simulink model "Motor_Control"  (R2020a)
settings: Solver=VariableStepAuto  StartTime=0.0  StopTime=2  RelTol=1e-3
values from neighbouring files (symbols this model uses):
  b = 2.58984 * 10^(-5)    (= 2.58984e-05)    [MotorInformation.m]
  d = 0.15    [MotorInformation.m]
  J = (1/12)*(0.32^2+0.4^2)*M + M*0.15^2    (= 0.354933333333)    [MotorInformation.m]
  Kac = 1/Kpc    (= 0.0636619772368)    [MotorInformation.m]
  Kas = 1/(2.8*Kps)    (= 40.4186448067)    [MotorInformation.m]
  Ke = 0.0195    [MotorInformation.m]
  Kic = R * Wcc*1.3    (= 24504.422698)    [MotorInformation.m]
  Kis = Jm*Wcs^2/(Kt)    (= 2.77594011786)    [MotorInformation.m]
  Kpc = La * Wcc    (= 15.7079632679)    [MotorInformation.m]
  Kps = Jm * Wcs/Kt    (= 0.00883609182968)    [MotorInformation.m]
  Kt = 0.0195    [MotorInformation.m]
  L = 0.1655    [MotorInformation.m]
  La = 0.005    [MotorInformation.m]
  M = 8    [MotorInformation.m]
  n = 49    [MotorInformation.m]
  R = 6    [MotorInformation.m]
  Rw = 0.155/2    (= 0.0775)    [MotorInformation.m]
libraries: simulink x2
settings Model: Creator=hambi  LastModifiedBy=hambi

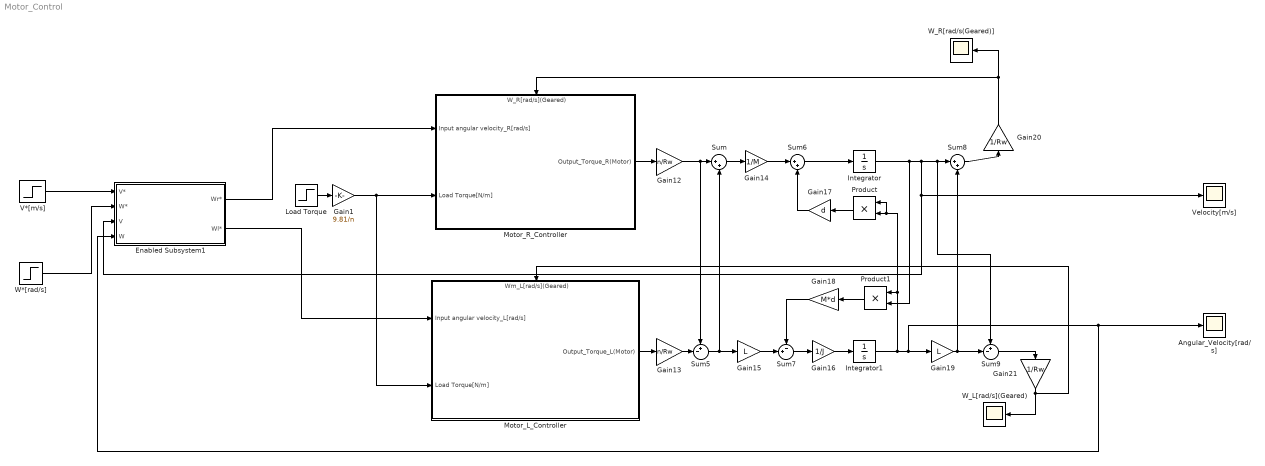
== system Motor_Control ==
  Angular_Velocity[rad/s] : Scope
  Enabled Subsystem1 : Subsystem  TreatAsAtomicUnit=on
  Gain1 : Gain  Gain=9.81/n
  Gain12 : Gain  Gain=n/Rw
  Gain13 : Gain  Gain=n/Rw
  Gain14 : Gain  Gain=1/M
  Gain15 : Gain  Gain=L
  Gain16 : Gain  Gain=1/J
  Gain17 : Gain  Gain=d
  Gain18 : Gain  Gain=M*d
  Gain19 : Gain  Gain=L
  Gain20 : Gain  Gain=1/Rw
  Gain21 : Gain  Gain=1/Rw
  Integrator : Integrator
  Integrator1 : Integrator
  Load Torque : Step  Time=5  After=0  SampleTime=0
  Motor_L_Controller : Subsystem  TreatAsAtomicUnit=on
      settings: PortSchema="{\"entries\":[{\"content\":{\"sides\":[{\"content\":{\"connectorIds\":[\"In1\",\"In2\"]},\"type\":\"ConnectorPlacement.EquallySpacedRectSide\",\"uuid\":\"38708cf0-fa5b-4525-8073-2ea034bbba89\"},{\"content\":{\"connectorIds\":[\"Out1\"],\"side\":\"RIGHT\"},\"type\":\"ConnectorPlacement.EquallySpacedRectSide\",\"uuid\":\"66c4a39b-21a9-4a0c-b844-f8b5c61f778e\"},{\"content\":{\"connectorIds\":[\"In3\"],\"side\":\"TOP\"},\"type\":\"ConnectorPlacement.EquallySpacedRectSide\",\"uuid\":\"4e6c23e5-8516-4ab2-b702-67db97948711\"}]},\"type\":\"ConnectorPlacement.EquallySpacedConnector\",\"uuid\":\"2dafcc4f-e74b-4b96-80e8-79cd761172ee\"}],\"packageUris\":[\"http://schema.mathworks.com/mf0/Connector/19700101\"],\"version\":\"1.0\"}"
  Motor_R_Controller : Subsystem  TreatAsAtomicUnit=on
      settings: PortSchema="{\"entries\":[{\"content\":{\"sides\":[{\"content\":{\"connectorIds\":[\"In1\",\"In2\"]},\"type\":\"ConnectorPlacement.EquallySpacedRectSide\",\"uuid\":\"38708cf0-fa5b-4525-8073-2ea034bbba89\"},{\"content\":{\"connectorIds\":[\"Out1\"],\"side\":\"RIGHT\"},\"type\":\"ConnectorPlacement.EquallySpacedRectSide\",\"uuid\":\"66c4a39b-21a9-4a0c-b844-f8b5c61f778e\"},{\"content\":{\"connectorIds\":[\"In3\"],\"side\":\"TOP\"},\"type\":\"ConnectorPlacement.EquallySpacedRectSide\",\"uuid\":\"4e6c23e5-8516-4ab2-b702-67db97948711\"}]},\"type\":\"ConnectorPlacement.EquallySpacedConnector\",\"uuid\":\"2dafcc4f-e74b-4b96-80e8-79cd761172ee\"}],\"packageUris\":[\"http://schema.mathworks.com/mf0/Connector/19700101\"],\"version\":\"1.0\"}"
  Product : Product
  Product1 : Product
  Sum : Sum  Inputs=|++
  Sum5 : Sum  Inputs=+-|
  Sum6 : Sum  Inputs=|++
  Sum7 : Sum  Inputs=-+|
  Sum8 : Sum  Inputs=|++
  Sum9 : Sum  Inputs=+-|
  V*[m/s] : Step  Time=0  After=0.20  SampleTime=0  ZeroCross=off
  Velocity[m/s] : Scope
  W*[rad/s] : Step  Time=0  After=0.028  SampleTime=0  ZeroCross=off
  W_L[rad/s](Geared) : Scope
  W_R[rad/s(Geared)] : Scope
  wires:
  Sum8/1 -> Gain20/1
  Gain20/1 -> Motor_R_Controller/3(W_R[rad/s](Geared)), W_R[rad/s(Geared)]/1
  Gain21/1 -> Motor_L_Controller/3(Wm_L[rad/s](Geared)), W_L[rad/s](Geared)/1
  Sum9/1 -> Gain21/1
  Product1/1 -> Gain18/1
  Product/1 -> Gain17/1
  Gain14/1 -> Sum6/1
  Gain16/1 -> Integrator1/1
  Motor_R_Controller/1(Output_Torque_R(Motor)) -> Gain12/1
  Integrator/1 -> Enabled Subsystem1/3(V), Velocity[m/s]/1, Sum9/1, Sum8/1, Product1/2
  Gain1/1 -> Motor_L_Controller/2(Load Torque[N/m]), Motor_R_Controller/2(Load Torque[N/m])
  Gain19/1 -> Sum9/2, Sum8/2
  Enabled Subsystem1/1(Wr*) -> Motor_R_Controller/1(Input angular velocity_R[rad/s])
  Motor_L_Controller/1(Output_Torque_L(Motor)) -> Gain13/1
  Gain13/1 -> Sum5/2
  Sum6/1 -> Integrator/1
  Sum7/1 -> Gain16/1
  Gain15/1 -> Sum7/2
  Gain18/1 -> Sum7/1
  Gain17/1 -> Sum6/2
  Gain12/1 -> Sum5/1, Sum/1
  Sum/1 -> Gain14/1
  Sum5/1 -> Gain15/1, Sum/2
  Load Torque/1 -> Gain1/1
  Integrator1/1 -> Angular_Velocity[rad/s]/1, Enabled Subsystem1/4(W), Gain19/1, Product/1, Product/2, Product1/1
  V*[m/s]/1 -> Enabled Subsystem1/1(V*)
  W*[rad/s]/1 -> Enabled Subsystem1/2(W*)
  Enabled Subsystem1/2(Wl*) -> Motor_L_Controller/1(Input angular velocity_L[rad/s])

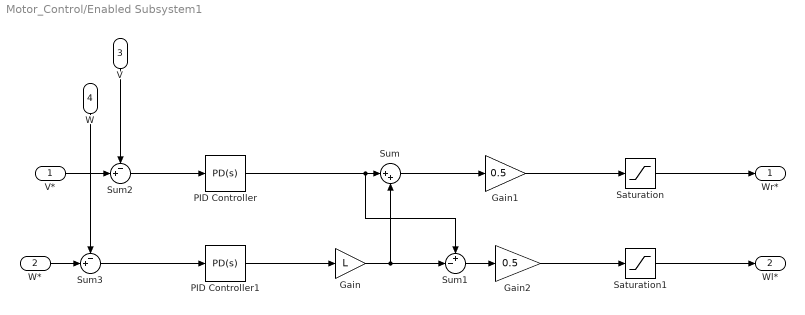
== system Motor_Control/Enabled Subsystem1 ==
  V* : Inport
  W* : Inport  Port=2
  V : Inport  Port=3
  W : Inport  Port=4
  Gain : Gain  Gain=L
  Gain1 : Gain  Gain=0.5
  Gain2 : Gain  Gain=0.5
  PID Controller : simulink/Continuous/PID Controller  Controller=PD  Form=Parallel  TimeDomain=Continuous-time  UseExternalTs=off  SampleTime=-1  IntegratorMethod=Forward Euler  FilterMethod=Forward Euler  ControllerParametersSource=internal  P=3.3  I=1  D=0.0145  UseFilter=on  N=100  TunerSelectOption=Transfer Function Based (PID Tuner App)  InitialConditionSource=internal  InitialConditionForIntegrator=0  InitialConditionForFilter=0  DifferentiatorICPrevScaledInput=0  ExternalReset=none  TrackingMode=off  Kt=1  LimitOutput=off  UpperSaturationLimit=inf  LowerSaturationLimit=-inf  LinearizeAsGain=on  AntiWindupMode=none  Kb=1  POutMin=[]  POutMax=[]  IOutMin=[]  IOutMax=[]  DOutMin=[]  DOutMax=[]  NOutMin=[]  NOutMax=[]  SumOutMin=[]  SumOutMax=[]  SaturationOutMin=[]  SaturationOutMax=[]  PParamMin=[]  PParamMax=[]  IParamMin=[]  IParamMax=[]  DParamMin=[]  DParamMax=[]  NParamMin=[]  NParamMax=[]  KbParamMin=[]  KbParamMax=[]  KtParamMin=[]  KtParamMax=[]  KbOutMin=[]  KbOutMax=[]  KtOutMin=[]  KtOutMax=[]  IntegratorOutMin=[]  IntegratorOutMax=[]  FilterOutMin=[]  FilterOutMax=[]  SumI1OutMin=[]  SumI1OutMax=[]  SumI2OutMin=[]  SumI2OutMax=[]  SumI3OutMin=[]  SumI3OutMax=[]  SumI4OutMin=[]  SumI4OutMax=[]  SumDOutMin=[]  SumDOutMax=[]  DifferentiatorOutMin=[]  DifferentiatorOutMax=[]  FilterDiffOutCoefMin=[]  FilterDiffOutCoefMax=[]  ReciprocalOutMin=[]  ReciprocalOutMax=[]  SumDenOutMin=[]  SumDenOutMax=[]  SumNumOutMin=[]  SumNumOutMax=[]  DivideOutMin=[]  DivideOutMax=[]  UdiffTsProdOutMin=[]  UdiffTsProdOutMax=[]  NTsProdOutMin=[]  NTsProdOutMax=[]  UintegralTsProdOutMin=[]  UintegralTsProdOutMax=[]  UngainTsProdOutMin=[]  UngainTsProdOutMax=[]  IntegratorContinuousStateAttributes=''  IntegratorStateMustResolveToSignalObject=off  IntegratorRTWStateStorageClass=Auto  FilterContinuousStateAttributes=''  FilterStateMustResolveToSignalObject=off  FilterRTWStateStorageClass=Auto  ParallelPVariant=InternalParameters  IdealPVariant=Disabled  IVariant=Disabled  DVariant=InternalParameters  IntegratorVariant=Disabled  SatVariant=Disabled  AWVariant=Disabled  PCopyVariant=Disabled  TRVariant=Disabled  FdbkBlocksVariant=Forward  IdealPFdbkVariant=Disabled  SatFdbkVariant=Disabled  DerivativeFilterVariant=ContFilter  NVariant=InternalParameters  NCopyVariant=Disabled  FilterICVariant=InternalICsFilter  IntegratorICVariant=Disabled  ExternalResetVariant=Disabled  TRSumVariant=Passthrough  SumFdbkVariant=Disabled  SumVariant=Sum_PD  TsampFilterVariant=InternalTs  TsampNgainVariant=Passthrough  TsampIntegralVariant=Disabled_SignalSpec
  PID Controller1 : simulink/Continuous/PID Controller  Controller=PD  Form=Parallel  TimeDomain=Continuous-time  UseExternalTs=off  SampleTime=-1  IntegratorMethod=Forward Euler  FilterMethod=Forward Euler  ControllerParametersSource=internal  P=5  I=1  D=0  UseFilter=on  N=100  TunerSelectOption=Transfer Function Based (PID Tuner App)  InitialConditionSource=internal  InitialConditionForIntegrator=0  InitialConditionForFilter=0  DifferentiatorICPrevScaledInput=0  ExternalReset=none  TrackingMode=off  Kt=1  LimitOutput=off  UpperSaturationLimit=inf  LowerSaturationLimit=-inf  LinearizeAsGain=on  AntiWindupMode=none  Kb=1  POutMin=[]  POutMax=[]  IOutMin=[]  IOutMax=[]  DOutMin=[]  DOutMax=[]  NOutMin=[]  NOutMax=[]  SumOutMin=[]  SumOutMax=[]  SaturationOutMin=[]  SaturationOutMax=[]  PParamMin=[]  PParamMax=[]  IParamMin=[]  IParamMax=[]  DParamMin=[]  DParamMax=[]  NParamMin=[]  NParamMax=[]  KbParamMin=[]  KbParamMax=[]  KtParamMin=[]  KtParamMax=[]  KbOutMin=[]  KbOutMax=[]  KtOutMin=[]  KtOutMax=[]  IntegratorOutMin=[]  IntegratorOutMax=[]  FilterOutMin=[]  FilterOutMax=[]  SumI1OutMin=[]  SumI1OutMax=[]  SumI2OutMin=[]  SumI2OutMax=[]  SumI3OutMin=[]  SumI3OutMax=[]  SumI4OutMin=[]  SumI4OutMax=[]  SumDOutMin=[]  SumDOutMax=[]  DifferentiatorOutMin=[]  DifferentiatorOutMax=[]  FilterDiffOutCoefMin=[]  FilterDiffOutCoefMax=[]  ReciprocalOutMin=[]  ReciprocalOutMax=[]  SumDenOutMin=[]  SumDenOutMax=[]  SumNumOutMin=[]  SumNumOutMax=[]  DivideOutMin=[]  DivideOutMax=[]  UdiffTsProdOutMin=[]  UdiffTsProdOutMax=[]  NTsProdOutMin=[]  NTsProdOutMax=[]  UintegralTsProdOutMin=[]  UintegralTsProdOutMax=[]  UngainTsProdOutMin=[]  UngainTsProdOutMax=[]  IntegratorContinuousStateAttributes=''  IntegratorStateMustResolveToSignalObject=off  IntegratorRTWStateStorageClass=Auto  FilterContinuousStateAttributes=''  FilterStateMustResolveToSignalObject=off  FilterRTWStateStorageClass=Auto  ParallelPVariant=InternalParameters  IdealPVariant=Disabled  IVariant=Disabled  DVariant=InternalParameters  IntegratorVariant=Disabled  SatVariant=Disabled  AWVariant=Disabled  PCopyVariant=Disabled  TRVariant=Disabled  FdbkBlocksVariant=Forward  IdealPFdbkVariant=Disabled  SatFdbkVariant=Disabled  DerivativeFilterVariant=ContFilter  NVariant=InternalParameters  NCopyVariant=Disabled  FilterICVariant=InternalICsFilter  IntegratorICVariant=Disabled  ExternalResetVariant=Disabled  TRSumVariant=Passthrough  SumFdbkVariant=Disabled  SumVariant=Sum_PD  TsampFilterVariant=InternalTs  TsampNgainVariant=Passthrough  TsampIntegralVariant=Disabled_SignalSpec
  Saturation : Saturate  UpperLimit=1.6  LowerLimit=-1.6
  Saturation1 : Saturate  UpperLimit=1.6  LowerLimit=-1.6
  Sum : Sum  Inputs=|++
  Sum1 : Sum  Inputs=+-|
  Sum2 : Sum  Inputs=-+|
  Sum3 : Sum  Inputs=-+|
  Wr* : Outport
  Wl* : Outport  Port=2
  wires:
  Gain/1 -> Sum1/2, Sum/2
  Sum/1 -> Gain1/1
  Sum1/1 -> Gain2/1
  Sum2/1 -> PID Controller/1
  W*/1 -> Sum3/2
  V/1 -> Sum2/1
  V*/1 -> Sum2/2
  W/1 -> Sum3/1
  Gain1/1 -> Saturation/1
  Gain2/1 -> Saturation1/1
  PID Controller/1 -> Sum1/1, Sum/1
  Sum3/1 -> PID Controller1/1
  PID Controller1/1 -> Gain/1
  Saturation/1 -> Wr*/1
  Saturation1/1 -> Wl*/1

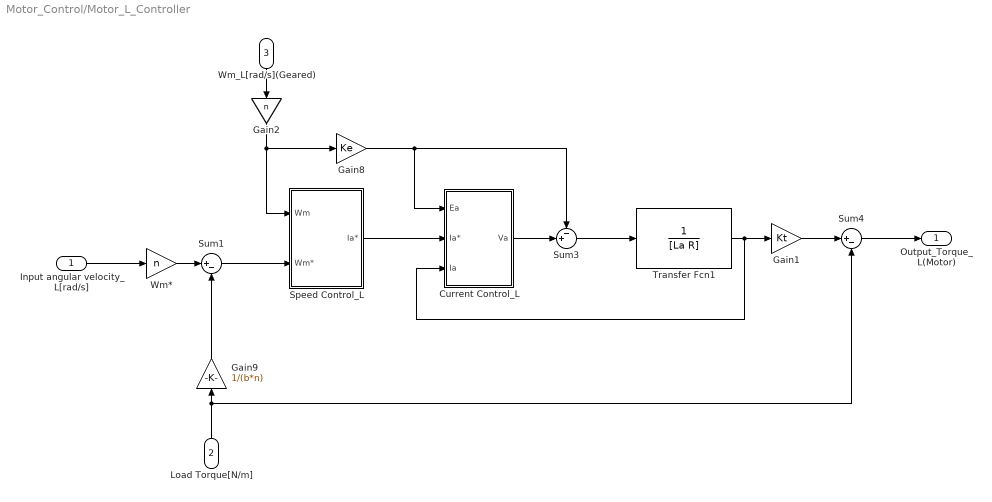
== system Motor_Control/Motor_L_Controller ==
  Input angular velocity_L[rad/s] : Inport
  Load Torque[N/m] : Inport  Port=2
  Wm_L[rad/s](Geared) : Inport  Port=3
  Current Control_L : Subsystem
  Gain1 : Gain  Gain=Kt
  Gain2 : Gain  Gain=n
  Gain8 : Gain  Gain=Ke
  Gain9 : Gain  Gain=1/(b*n)
  Speed Control_L : Subsystem
  Sum1 : Sum  Inputs=|+-
  Sum3 : Sum  Inputs=-+|
  Sum4 : Sum  Inputs=|+-
  Transfer Fcn1 : TransferFcn  Denominator=[La R]
  Wm* : Gain  Gain=n
  Output_Torque_L(Motor) : Outport
  wires:
  Input angular velocity_L[rad/s]/1 -> Wm*/1
  Sum1/1 -> Speed Control_L/2(Wm*)
  Speed Control_L/1(Ia*) -> Current Control_L/2(Ia*)
  Gain9/1 -> Sum1/2
  Load Torque[N/m]/1 -> Sum4/2, Gain9/1
  Wm*/1 -> Sum1/1
  Transfer Fcn1/1 -> Current Control_L/3(Ia), Gain1/1
  Current Control_L/1(Va) -> Sum3/2
  Sum3/1 -> Transfer Fcn1/1
  Gain8/1 -> Sum3/1, Current Control_L/1(Ea)
  Gain1/1 -> Sum4/1
  Sum4/1 -> Output_Torque_L(Motor)/1
  Gain2/1 -> Gain8/1, Speed Control_L/1(Wm)
  Wm_L[rad/s](Geared)/1 -> Gain2/1

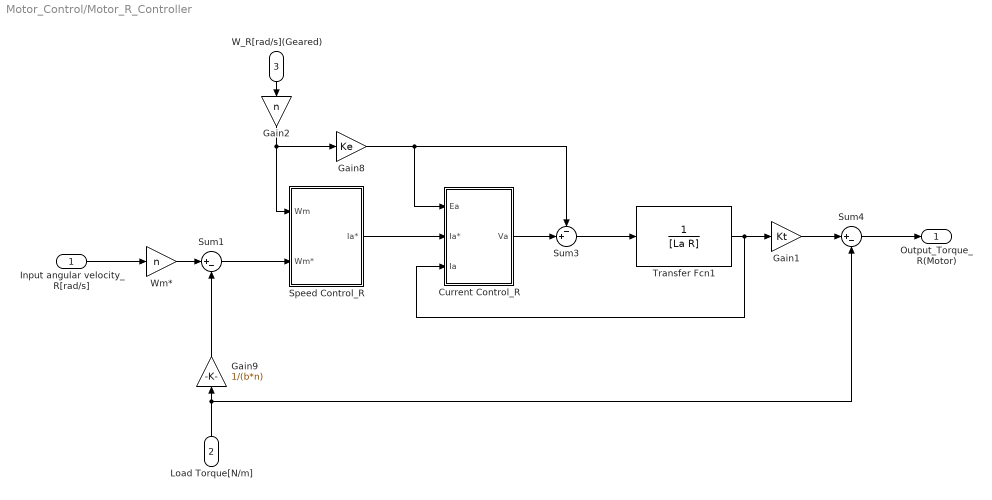
== system Motor_Control/Motor_R_Controller ==
  Input angular velocity_R[rad/s] : Inport
  Load Torque[N/m] : Inport  Port=2
  W_R[rad/s](Geared) : Inport  Port=3
  Current Control_R : Subsystem
  Gain1 : Gain  Gain=Kt
  Gain2 : Gain  Gain=n
  Gain8 : Gain  Gain=Ke
  Gain9 : Gain  Gain=1/(b*n)
  Speed Control_R : Subsystem
  Sum1 : Sum  Inputs=|+-
  Sum3 : Sum  Inputs=-+|
  Sum4 : Sum  Inputs=|+-
  Transfer Fcn1 : TransferFcn  Denominator=[La R]
  Wm* : Gain  Gain=n
  Output_Torque_R(Motor) : Outport
  wires:
  Input angular velocity_R[rad/s]/1 -> Wm*/1
  Sum1/1 -> Speed Control_R/2(Wm*)
  Speed Control_R/1(Ia*) -> Current Control_R/2(Ia*)
  Gain9/1 -> Sum1/2
  Load Torque[N/m]/1 -> Sum4/2, Gain9/1
  Wm*/1 -> Sum1/1
  Transfer Fcn1/1 -> Current Control_R/3(Ia), Gain1/1
  Current Control_R/1(Va) -> Sum3/2
  Sum3/1 -> Transfer Fcn1/1
  Gain8/1 -> Sum3/1, Current Control_R/1(Ea)
  Gain1/1 -> Sum4/1
  Sum4/1 -> Output_Torque_R(Motor)/1
  W_R[rad/s](Geared)/1 -> Gain2/1
  Gain2/1 -> Speed Control_R/1(Wm), Gain8/1

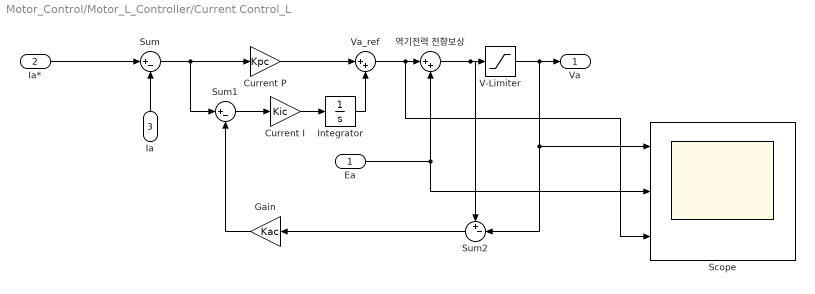
== system Motor_Control/Motor_L_Controller/Current Control_L ==
  Ea : Inport
  Ia* : Inport  Port=2
  Ia : Inport  Port=3
  Current I : Gain  Gain=Kic
  Current P : Gain  Gain=Kpc
  Gain : Gain  Gain=Kac
  Integrator : Integrator
  Scope : Scope  NumInputPorts=3
  Sum : Sum  Inputs=|+-
  Sum1 : Sum  Inputs=|+-
  Sum2 : Sum  Inputs=+-|
  V-Limiter : Saturate  UpperLimit=12  LowerLimit=-12  ZeroCross=off
  Va_ref : Sum  Inputs=|++
  역기전력 전향보상 : Sum  Inputs=|++
  Va : Outport
  wires:
  Integrator/1 -> Va_ref/2
  Current P/1 -> Va_ref/1
  Sum/1 -> Current P/1, Sum1/1
  Current I/1 -> Integrator/1
  Va_ref/1 -> Scope/3, 역기전력 전향보상/1
  Ia/1 -> Sum/2
  Ia*/1 -> Sum/1
  역기전력 전향보상/1 -> Sum2/1, V-Limiter/1
  V-Limiter/1 -> Scope/1, Sum2/2, Va/1
  Sum1/1 -> Current I/1
  Gain/1 -> Sum1/2
  Sum2/1 -> Gain/1
  Ea/1 -> Scope/2, 역기전력 전향보상/2

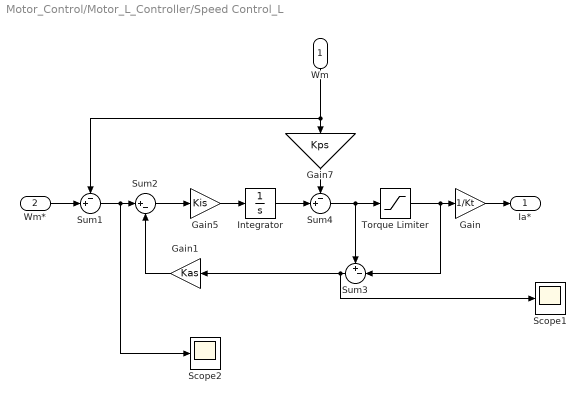
== system Motor_Control/Motor_L_Controller/Speed Control_L ==
  Wm : Inport
  Wm* : Inport  Port=2
  Gain : Gain  Gain=1/Kt
  Gain1 : Gain  Gain=Kas
  Gain5 : Gain  Gain=Kis
  Gain7 : Gain  Gain=Kps
  Integrator : Integrator
  Scope1 : Scope
  Scope2 : Scope
  Sum1 : Sum  Inputs=-+|
  Sum2 : Sum  Inputs=|+-
  Sum3 : Sum  Inputs=+-|
  Sum4 : Sum  Inputs=-+|
  Torque Limiter : Saturate  UpperLimit=999999  LowerLimit=-999999  ZeroCross=off
  Ia* : Outport
  wires:
  Gain7/1 -> Sum4/1
  Gain5/1 -> Integrator/1
  Integrator/1 -> Sum4/2
  Gain/1 -> Ia*/1
  Wm*/1 -> Sum1/2
  Wm/1 -> Sum1/1, Gain7/1
  Sum4/1 -> Sum3/1, Torque Limiter/1
  Torque Limiter/1 -> Sum3/2, Gain/1
  Sum3/1 -> Scope1/1, Gain1/1
  Gain1/1 -> Sum2/2
  Sum1/1 -> Scope2/1, Sum2/1
  Sum2/1 -> Gain5/1

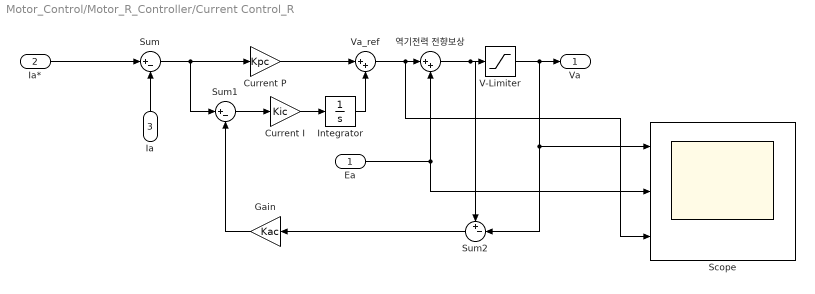
== system Motor_Control/Motor_R_Controller/Current Control_R ==
  Ea : Inport
  Ia* : Inport  Port=2
  Ia : Inport  Port=3
  Current I : Gain  Gain=Kic
  Current P : Gain  Gain=Kpc
  Gain : Gain  Gain=Kac
  Integrator : Integrator
  Scope : Scope  NumInputPorts=3
  Sum : Sum  Inputs=|+-
  Sum1 : Sum  Inputs=|+-
  Sum2 : Sum  Inputs=+-|
  V-Limiter : Saturate  UpperLimit=12  LowerLimit=-12  ZeroCross=off
  Va_ref : Sum  Inputs=|++
  역기전력 전향보상 : Sum  Inputs=|++
  Va : Outport
  wires:
  Integrator/1 -> Va_ref/2
  Current P/1 -> Va_ref/1
  Sum/1 -> Current P/1, Sum1/1
  Current I/1 -> Integrator/1
  Va_ref/1 -> Scope/3, 역기전력 전향보상/1
  Ia/1 -> Sum/2
  Ia*/1 -> Sum/1
  역기전력 전향보상/1 -> Sum2/1, V-Limiter/1
  V-Limiter/1 -> Scope/1, Sum2/2, Va/1
  Sum1/1 -> Current I/1
  Gain/1 -> Sum1/2
  Sum2/1 -> Gain/1
  Ea/1 -> Scope/2, 역기전력 전향보상/2

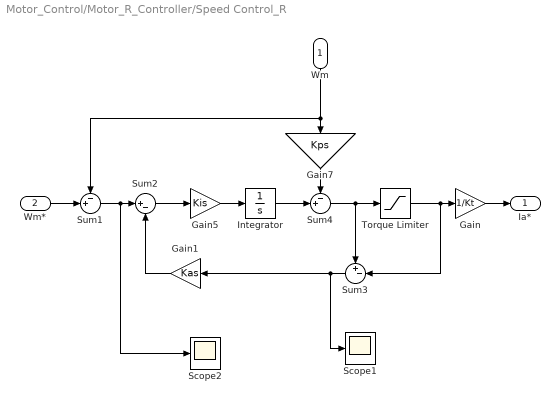
== system Motor_Control/Motor_R_Controller/Speed Control_R ==
  Wm : Inport
  Wm* : Inport  Port=2
  Gain : Gain  Gain=1/Kt
  Gain1 : Gain  Gain=Kas
  Gain5 : Gain  Gain=Kis
  Gain7 : Gain  Gain=Kps
  Integrator : Integrator
  Scope1 : Scope
  Scope2 : Scope
  Sum1 : Sum  Inputs=-+|
  Sum2 : Sum  Inputs=|+-
  Sum3 : Sum  Inputs=+-|
  Sum4 : Sum  Inputs=-+|
  Torque Limiter : Saturate  UpperLimit=999999  LowerLimit=-999999  ZeroCross=off
  Ia* : Outport
  wires:
  Gain7/1 -> Sum4/1
  Gain5/1 -> Integrator/1
  Integrator/1 -> Sum4/2
  Gain/1 -> Ia*/1
  Wm*/1 -> Sum1/2
  Wm/1 -> Sum1/1, Gain7/1
  Sum4/1 -> Sum3/1, Torque Limiter/1
  Torque Limiter/1 -> Sum3/2, Gain/1
  Sum3/1 -> Scope1/1, Gain1/1
  Gain1/1 -> Sum2/2
  Sum1/1 -> Scope2/1, Sum2/1
  Sum2/1 -> Gain5/1
